simulink model "channel_sfunc"  (R2020b)
settings: Solver=VariableStepAuto  StartTime=0.0  StopTime=10.0  RelTol=1e-3
libraries: dspsrcs4 x2, commchan3 x1, simulink_extras x1, commsink2 x1, commfilt2 x1, commrandsrc3 x1, dspsigops x1
settings Model: Creator=Yogapriya  LastModifiedBy=Yogapriya

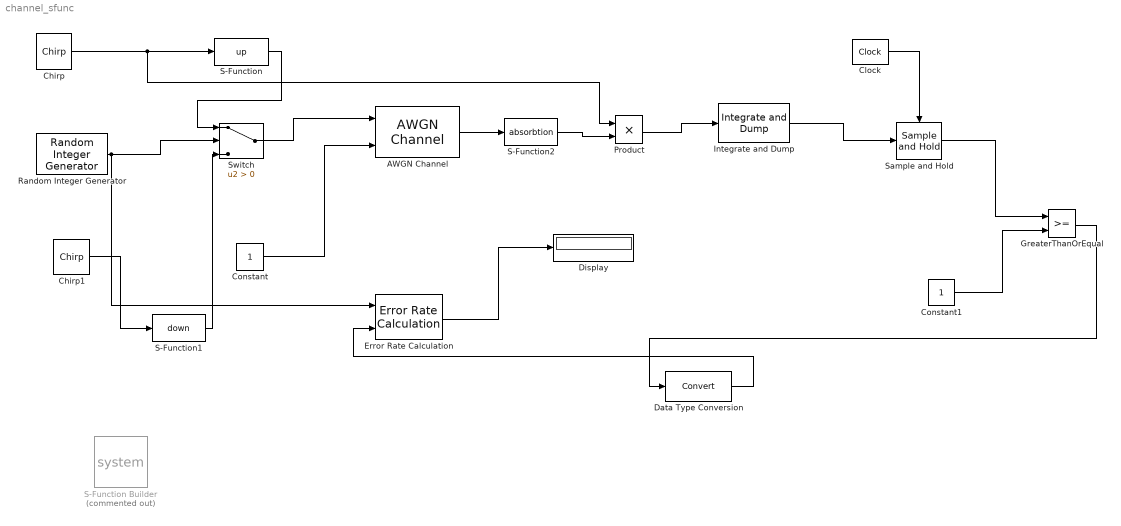
== system channel_sfunc ==
  AWGN Channel : commchan3/AWGN Channel  InputProcessing=Columns as channels (frame based)  seed=67  noiseMode=Variance from port  EbNodB=10  EsNodB=10  SNRdB=10  bitsPerSym=1  Ps=1  Tsym=1  variance=1
  Chirp : dspsrcs4/Chirp  sweep=Linear  mode=Unidirectional  f0=1000  f1=4000  t1=1  Tsweep=1  phase=0  Ts=1/8000  spf=1  datatype=Double  OutputFrames=off
  Chirp1 : dspsrcs4/Chirp  sweep=Linear  mode=Unidirectional  f0=1000  f1=4000  t1=1  Tsweep=1  phase=0  Ts=1/8000  spf=1  datatype=Double  OutputFrames=off
  Clock : simulink_extras/Flip Flops/Clock  period=2
  Constant : Constant
  Constant1 : Constant
  Data Type Conversion : DataTypeConversion
  Display : Display
  Error Rate Calculation : commsink2/Error Rate Calculation  N=0  st_delay=0  cp_mode=Entire frame  subframe=[]  PMode=Port  WsName=ErrorVec  RsMode2=off  stop=off  numErr=100  maxBits=1e6
  GreaterThanOrEqual : RelationalOperator  OutDataTypeStr=boolean  RndMeth=Simplest
  Integrate and Dump : commfilt2/Integrate and Dump  obssamples=8  offsetsamples=0  nodump=off  roundingMode=Floor  overflowMode=off  outputDataTypeStr=Inherit: Same as accumulator  outputLastDataTypeStr=Inherit: Same as accumulator
  Product : Product
  Random Integer Generator : commrandsrc3/Random Integer Generator  SetSize=8  SeedSource=Auto  Seed=0  SampleTime=1  SamplesPerFrame=1  OutputDataType=double  SimulateUsing=Interpreted execution
  S-Function : S-Function  FunctionName=up  SFunctionDeploymentMode=off  EnableBusSupport=off
  S-Function Builder : S-Function  Commented=on  SFunctionDeploymentMode=off  EnableBusSupport=off  mask(S-Function Builder){}
      mask help: Simulink:masks:SFunctionBuilder_MD
      mask init:
      | val = [[.9  0.75 0.75 1 1 .9 .9 1]',[1 1 0.75 0.75 .9 .9 1 .9]'];
      | sys = get_param(gcbh,'FunctionName');
      settings: CopyFcn=set_param(gcbh,'LinkStatus','none')  OpenFcn=sfunctionwizard(gcbh)
      mask Display:
      | plot(val(:,1),val(:,2))
      | disp(sys)
  S-Function1 : S-Function  FunctionName=down  SFunctionDeploymentMode=off  EnableBusSupport=off
  S-Function2 : S-Function  FunctionName=absorbtion  SFunctionDeploymentMode=off  EnableBusSupport=off
  Sample and Hold : dspsigops/Sample and Hold  trig=Rising edge  initCond=0  latchinput=off
  Switch : Switch  Criteria=u2 > Threshold
  wires:
  Constant/1 -> AWGN Channel/2
  Switch/1 -> AWGN Channel/1
  AWGN Channel/1 -> S-Function2/1
  Chirp/1 -> Product/1, S-Function/1
  S-Function/1 -> Switch/1
  Chirp1/1 -> S-Function1/1
  S-Function1/1 -> Switch/3
  S-Function2/1 -> Product/2
  Product/1 -> Integrate and Dump/1
  Integrate and Dump/1 -> Sample and Hold/1
  Clock/1 -> Sample and Hold/Trigger
  Sample and Hold/1 -> GreaterThanOrEqual/1
  Constant1/1 -> GreaterThanOrEqual/2
  GreaterThanOrEqual/1 -> Data Type Conversion/1
  Data Type Conversion/1 -> Error Rate Calculation/2
  Random Integer Generator/1 -> Error Rate Calculation/1, Switch/2
  Error Rate Calculation/1 -> Display/1
